simulink model "DirectedEvent5_2018a"  (R2018a)
settings: Solver=VariableStepAuto  StartTime=0.0  StopTime=0.1  RelTol=1e-3
settings Model: Creator=86188  LastModifiedBy=bzhan

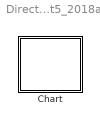
== system DirectedEvent5_2018a ==
  Chart : Stateflow chart  TreatAsAtomicUnit=on

== stateflow chart DirectedEvent5_2018a/Chart ==
  settings: updateMethod=DISCRETE  sampleTime=0.1
  state AM
    state A [parallel]
      settings: executionOrder=1
      state A2
        en: f("en_A2")
        ex: f("ex_A2")
      state A1
        en: f("en_A1")
        ex: f("ex_A1")
      (default) -> A1
      A1 -> A2 : [data==1]{send(E_one,B.B1.B2)}
      A2 -> A1 : E_two
    state B [parallel]
      settings: executionOrder=2
      state B1
        state B2
          en: f("en_B2")
          ex: f("ex_B2")
          state B21
            en: f("en_B21")
            ex: f("ex_B21")
          state B22
            en: f("en_B22")
            ex: f("ex_B22")
          (default) -> B21
          B21 -> B22 : E_one
        state B3
          en: f("en_B2")
          ex: f("ex_B2")
        (default) -> B2
        B2 -> B3 : E_two
        B3 -> B2 : E_one
      state B4
        en: f("en_B4")
        ex: f("ex_B4")
      (default) -> B1
      B1 -> B4 : E_one
      B4 -> B1 : E_two
  (default) -> AM
  data: s function_input; data local =1
  events: E_one local FUNCTION_CALL_EVENT; E_two local FUNCTION_CALL_EVENT
  function f(s):
    | function f(s)
    |   fprintf(s+"\n");
